simulink model "Boeing737Sample_updatedCopy"  (Simulink 8.2)
settings: Solver=ode45  StartTime=0.0  StopTime=100  RelTol=1e-3
InitFcn:
  | load('loss_coeff_mixing_junction.mat')
  | %load('defaultMSSN.mat')
  | load('SampleOutput.mat')
  | load('HydProp.mat')
  | load('HydraulicLoad.mat')
  | load('initavload.mat')
  | %load('mission_short.mat')
values from neighbouring files (symbols this model uses):
  avload =     [Benchmark_data1.mat]
  FuelBurn = [0 0 0 0 0 0 0 0 0 0 0 0 ... (18249 elements, 1x18249)]    [Benchmark_data1.mat]
undefined symbols (not defined in the file or in its folder): ailerons, B_737, elevator, F1, F2, HUGHES_TREITLER, landing_gear, PN_70147, rudder, thrust_rev
libraries: PowerFlowLib x91, simulink x19
(part 1 of 8)
settings Model: Creator=mwillms4  LastModifiedBy=srikanthan
settings DebuggingCC: FcnCallInpInsideContextMsg=EnableAllAsWarning  UnconnectedInputMsg=none  UnconnectedOutputMsg=none  UnconnectedLineMsg=none

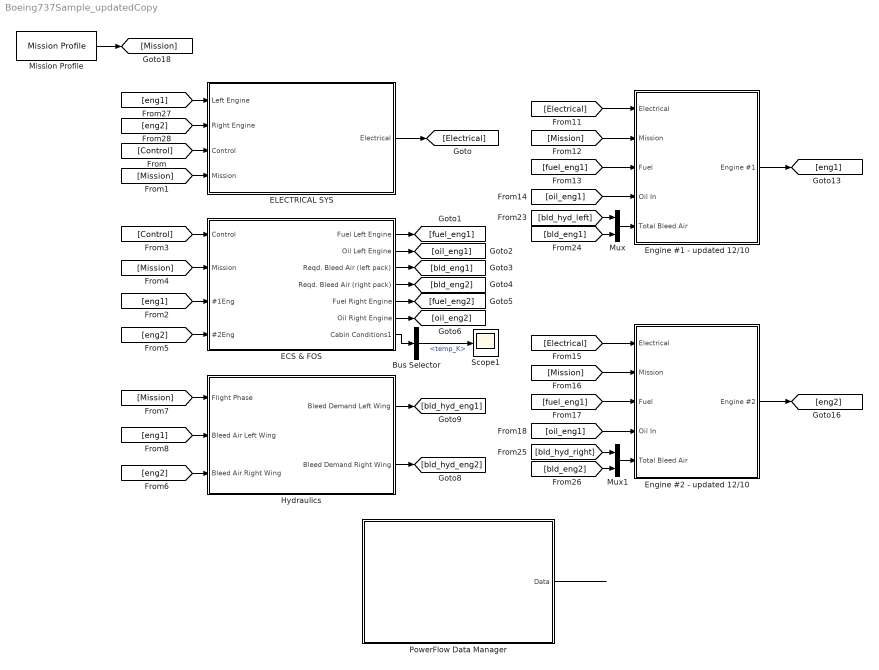
== system Boeing737Sample_updatedCopy ==
  Bus Selector : BusSelector  OutputSignals=temp_K
  "ECS & FOS " : Subsystem
  "ELECTRICAL SYS " : Subsystem
  Engine #1 - updated 12/10 : Subsystem
  Engine #2 - updated 12/10 : Subsystem
  "Hydraulics " : Subsystem
  Mission Profile : PowerFlowLib/Mission Profile/Mission Profile  mssn_check=off  mssn_prof=MSSN  del_P=0  del_T=0  del_rho=0  pres_msl=101.3  temp_msl=15  dens_msl=1.229
  Mux : Mux  Inputs=2
  Mux1 : Mux  Inputs=2
  PowerFlow Data Manager : Subsystem  AncestorBlock=PowerFlowLib/Support Functions//Tools/PowerFlow Data Manager
      mask init:
      | set_param(gcb, 'LinkStatus', 'inactive')    % disable the library link
      settings: OpenFcn=data_manager
      mask Display: str ='PowerFlow Data Manager\n(Double click to select variables for output)'; fprintf(str)
  Scope1 : Scope
      settings: YMin=295.065  YMax=295.075  SaveName=ScopeData36
  wires:
  Mission Profile/1 -> [Mission]
  "ELECTRICAL SYS "/1(Electrical) -> [Electrical]
  Engine #1 - updated 12/10/1(Engine #1) -> [eng1]
  Engine #2 - updated 12/10/1(Engine #2) -> [eng2]
  "Hydraulics "/2(Bleed Demand Right Wing) -> [bld_hyd_eng2]
  "Hydraulics "/1(Bleed Demand Left Wing) -> [bld_hyd_eng1]
  "ECS & FOS "/1("Fuel Left Engine ") -> [fuel_eng1]
  "ECS & FOS "/2(Oil Left Engine) -> [oil_eng1]
  "ECS & FOS "/3(Reqd. Bleed Air (left pack)) -> [bld_eng1]
  "ECS & FOS "/4(Reqd. Bleed Air (right pack)) -> [bld_eng2]
  "ECS & FOS "/5(Fuel Right Engine) -> [fuel_eng2]
  "ECS & FOS "/6(Oil Right Engine) -> [oil_eng2]
  [Mission] -> "Hydraulics "/1(Flight Phase)
  [eng2] -> "Hydraulics "/3(Bleed Air Right Wing)
  [eng1] -> "Hydraulics "/2(Bleed Air Left Wing)
  [Control] -> "ECS & FOS "/1(Control)
  [Mission] -> "ECS & FOS "/2(Mission)
  [Electrical] -> Engine #1 - updated 12/10/1(Electrical)
  [Mission] -> Engine #1 - updated 12/10/2(Mission)
  [fuel_eng1] -> Engine #1 - updated 12/10/3(Fuel)
  [oil_eng1] -> Engine #1 - updated 12/10/4(Oil In)
  [Electrical] -> Engine #2 - updated 12/10/1(Electrical)
  [Mission] -> Engine #2 - updated 12/10/2(Mission)
  [fuel_eng1] -> Engine #2 - updated 12/10/3(Fuel)
  [oil_eng1] -> Engine #2 - updated 12/10/4(Oil In)
  Mux/1 -> Engine #1 - updated 12/10/5(Total Bleed Air)
  [bld_eng1] -> Mux/2
  [bld_hyd_left] -> Mux/1
  Mux1/1 -> Engine #2 - updated 12/10/5(Total Bleed Air)
  [bld_eng2] -> Mux1/2
  [bld_hyd_right] -> Mux1/1
  Bus Selector/1 -> Scope1/1  "<temp_K>"
  [eng1] -> "ECS & FOS "/3(#1Eng)
  [eng2] -> "ECS & FOS "/4(#2Eng)
  PowerFlow Data Manager/1(Data) -> ?
  [Control] -> "ELECTRICAL SYS "/3(Control)
  [eng1] -> "ELECTRICAL SYS "/1(Left Engine)
  [eng2] -> "ELECTRICAL SYS "/2(Right Engine)
  [Mission] -> "ELECTRICAL SYS "/4(Mission)
  "ECS & FOS "/7(Cabin Conditions1) -> Bus Selector/1

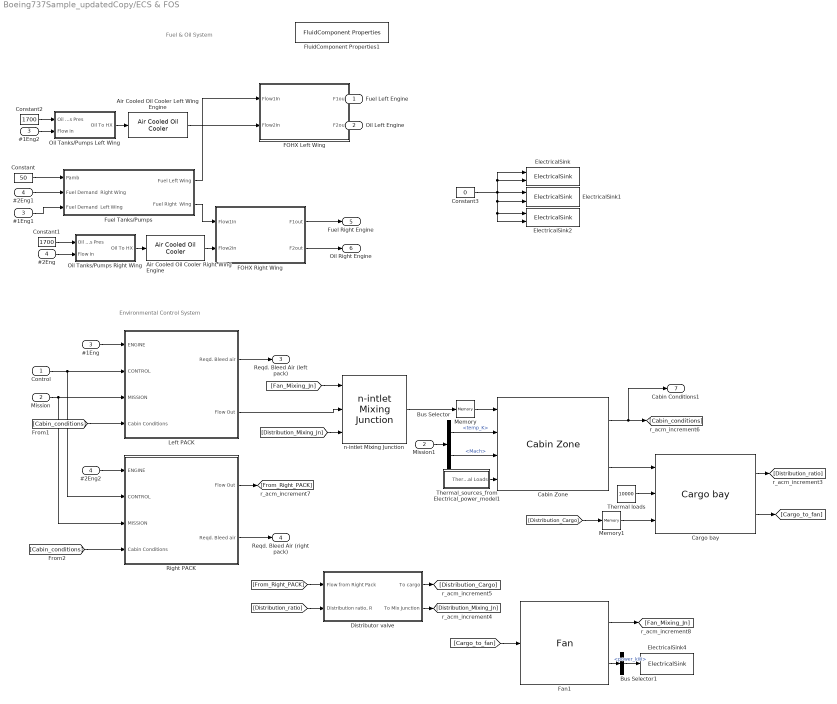
== system Boeing737Sample_updatedCopy/ECS & FOS  ==
  note: Environmental Control System
  note: Fuel & Oil System
  Control : Inport
  Mission : Inport  Port=2
  #1Eng : Inport  Port=3
  #2Eng : Inport  Port=4
  #1Eng1 : InportShadow  Port=3
  #1Eng2 : InportShadow  Port=3
  #2Eng1 : InportShadow  Port=4
  #2Eng2 : InportShadow  Port=4
  Air Cooled Oil Cooler Left Wing Engine : PowerFlowLib/Energy & Power Systems/Thermal/Oil/Air Cooled Oil Cooler  fileslct=off  filename=HeatExchangers.mat  filedir=C:\Users\mwillms4\Dropbox\School\Graduate\Research\PowerFlow Summer 2013\PropertyTables\HeatExchangers.mat  refresh=off  hx=HUGHES_TREITLER - PN_70147  bypass_full=1  bypass_none=100  hx_delP=82.74  hx_P=2068  hx_Qdot=24.27  hx_Vdot=0.000505  hx_mass=4.42
  Air Cooled Oil Cooler Right Wing Engine : PowerFlowLib/Energy & Power Systems/Thermal/Oil/Air Cooled Oil Cooler  fileslct=off  filename=HeatExchangers.mat  filedir=C:\Users\mwillms4\Dropbox\School\Graduate\Research\PowerFlow Summer 2013\PropertyTables\HeatExchangers.mat  refresh=off  hx=HUGHES_TREITLER - PN_70147  bypass_full=1  bypass_none=100  hx_delP=82.74  hx_P=2068  hx_Qdot=24.27  hx_Vdot=0.000505  hx_mass=4.42
  Bus Selector : BusSelector  OutputSignals=Flight parameters.temp_K,Flight parameters.Mach
  Bus Selector1 : BusSelector  OutputSignals=power_kW
  Cabin Zone : PowerFlowLib/Energy & Power Systems/Thermal/ECS/Cabin Zone  A_fuselage=320  V_cab=130.3  n_pass=176  L_shell=0.003  K_shell=1  L_insulation=0.02  K_insulation=1  L_coating=0.002  K_coating=1  Vdot_sa_pass=0.009438  q_pass=60  RAR=.25  h_outside=1  h_inside=1
  Cargo bay : PowerFlowLib/Energy & Power Systems/Thermal/ECS/Cargo bay  T_cargo_K=305
  Constant : Constant  Value=50
  Constant1 : Constant  Value=1700
  Constant2 : Constant  Value=1700
  Constant3 : Constant  Value=0
  Distributor valve : Subsystem
  ElectricalSink : PowerFlowLib/Support Functions//Tools/ElectricalSink  Tag=Flow  Description=TwoPhase  load_loc=Empennage  ACDC_load=AC  units=Kilowatts  unq_id=6691
  ElectricalSink1 : PowerFlowLib/Support Functions//Tools/ElectricalSink  Tag=Flow  Description=TwoPhase  load_loc=Cagobay  ACDC_load=AC  units=Kilowatts  unq_id=1878
  ElectricalSink2 : PowerFlowLib/Support Functions//Tools/ElectricalSink  Tag=Flow  Description=TwoPhase  load_loc=Cabin  ACDC_load=AC  units=Kilowatts  unq_id=3506
  ElectricalSink4 : PowerFlowLib/Support Functions//Tools/ElectricalSink  Tag=Flow  Description=TwoPhase  load_loc=Cabin  ACDC_load=DC  units=Kilowatts  unq_id=8332
  FOHX Left Wing : Subsystem  Description=TwoPhase  mask{fld1=JP8, fld2=LubeOil7808, alpha1=80, alpha2=80, N1=10, N2=10, A1_c=.1, A2_c=.1, A1_s=.25, A2_s=.25, P1init=620.5, P2init=620.5}
      mask prompts: fld1 "Fluid 1 Type"; fld2 "Fluid 2 Type"; alpha1 "Fluid 1 HTC [W/m² K]"; alpha2 "Fluid 2 HTC [W/m² K]"; N1 "Flow 1: Number of Channels"; N2 "Flow 2: Number of Channels"; A1_c "Flow 1: Cross-sectional area [m^2]"; A2_c "Flow 2: Cross-sectional area [m^2]"; A1_s "Flow 1: Total surface area [m^2]"; A2_s "Flow 2: Total surface area [m^2]"; P1init "Flow 1 Pressure [kPa]"; P2init "Flow 2 Pressure [kPa]"
      mask init:
      | %load TMSFluidProperties
      | %eval(['SF = FluidProp.SinglePhase.' get_param(gcb,'fld_type1') ';']);
      | %eval(['F = FluidProp.TwoPhase.' get_param(gcb,'fld_type2') ';']);
      | %FluidProp = FluidProp.TwoPhase.R134a; 
      | %{
      | if strcmp(get_param(bdroot,'SimulationStatus'),'initializing') ;
      |     load TwoPhaseProp_Evap
      |     TwoPhaseProp = TwoPhaseProp_Evap;
      |     Evaporator_Init_AFRL;
      | end
      | TMS_SetPhysSigs
      | if strcmp(get_param(gcb,'fld_type1'),'MoistAir')
      |     notair = 0 ; 
      | else
      |     notair = 1 ;
      | end
      | %}
      mask TypeOptions fld1: JP8
      mask TypeOptions fld2: LubeOil7808
      mask Display:
      | port_label('input',1,'Fuel In','TexMode','on') ;
      | port_label('input',2,'Oil In','TexMode','on') ;
      | port_label('output',1,'Fuel Out','TexMode','on') ;
      | port_label('output',2,'Oil Out','TexMode','on') ;
  FOHX Right Wing : Subsystem  Description=TwoPhase  mask{fld1=JP8, fld2=LubeOil7808, alpha1=80, alpha2=80, N1=10, N2=10, A1_c=.1, A2_c=.1, A1_s=.25, A2_s=.25, P1init=620.5, P2init=620.5}
      mask prompts: fld1 "Fluid 1 Type"; fld2 "Fluid 2 Type"; alpha1 "Fluid 1 HTC [W/m² K]"; alpha2 "Fluid 2 HTC [W/m² K]"; N1 "Flow 1: Number of Channels"; N2 "Flow 2: Number of Channels"; A1_c "Flow 1: Cross-sectional area [m^2]"; A2_c "Flow 2: Cross-sectional area [m^2]"; A1_s "Flow 1: Total surface area [m^2]"; A2_s "Flow 2: Total surface area [m^2]"; P1init "Flow 1 Pressure [kPa]"; P2init "Flow 2 Pressure [kPa]"
      mask init: same as Boeing737Sample_updatedCopy/ECS & FOS /FOHX Left Wing
      mask TypeOptions fld1: JP8
      mask TypeOptions fld2: LubeOil7808
      mask Display:
      | port_label('input',1,'Fuel In','TexMode','on') ;
      | port_label('input',2,'Oil In','TexMode','on') ;
      | port_label('output',1,'Fuel Out','TexMode','on') ;
      | port_label('output',2,'Oil Out','TexMode','on') ;
  Fan1 : PowerFlowLib/Energy & Power Systems/Thermal/ECS/Fan  N_fan=1725
  FluidComponent Properties1 : PowerFlowLib/Support Functions//Tools/FluidComponent Properties  fuelprop=FluidProp_JetA3638.mat  oilprop=OilProp.mat  airprop=AirProp.mat  pumpprop=PumpProp.mat  fanprop=Fanmap.mat  compprop=CompProp.mat  heatexprop=HeatExchangers.mat
  Fuel Tanks/Pumps : Subsystem
  Left PACK : Subsystem
  Memory : Memory
  Memory1 : Memory
  Mission1 : InportShadow  Port=2
  Oil Tanks/Pumps Left Wing : Subsystem
  Oil Tanks/Pumps Right Wing : Subsystem
  Right PACK : Subsystem
  Thermal loads : Constant  Value=10000
  Thermal_sources_from Electrical_power_model1 : Subsystem
  n-intlet Mixing Junction : PowerFlowLib/Energy & Power Systems/Thermal/ECS/n-intlet Mixing Junction  no_inlets=3  d_in_1=0.1  d_in_2=0.1  d_out=0.2
  "Fuel Left Engine " : Outport
  Oil Left Engine : Outport  Port=2
  Reqd. Bleed Air (left pack) : Outport  Port=3
  Reqd. Bleed Air (right pack) : Outport  Port=4
  Fuel Right Engine : Outport  Port=5
  Oil Right Engine : Outport  Port=6
  Cabin Conditions1 : Outport  Port=7
  wires:
  Left PACK/1(Reqd. Bleed air) -> Reqd. Bleed Air (left pack)/1
  Control/1 -> Left PACK/2(CONTROL), Right PACK/2(CONTROL)
  Mission/1 -> Left PACK/3(MISSION), Right PACK/3(MISSION)
  Right PACK/2(Reqd. Bleed air) -> Reqd. Bleed Air (right pack)/1
  Constant/1 -> Fuel Tanks/Pumps/1(Pamb)
  Air Cooled Oil Cooler Right Wing Engine/1 -> FOHX Right Wing/2(Flow2In)
  Fuel Tanks/Pumps/2(Fuel Right  Wing) -> FOHX Right Wing/1(Flow1In)
  Oil Tanks/Pumps Right Wing/1(Oil To HX) -> Air Cooled Oil Cooler Right Wing Engine/1
  Constant1/1 -> Oil Tanks/Pumps Right Wing/1(Oil Sys Pres)
  FOHX Right Wing/1(F1out) -> Fuel Right Engine/1
  Air Cooled Oil Cooler Left Wing Engine/1 -> FOHX Left Wing/2(Flow2In)
  Oil Tanks/Pumps Left Wing/1(Oil To HX) -> Air Cooled Oil Cooler Left Wing Engine/1
  Constant2/1 -> Oil Tanks/Pumps Left Wing/1(Oil Sys Pres)
  Fuel Tanks/Pumps/1(Fuel Left Wing) -> FOHX Left Wing/1(Flow1In)
  FOHX Left Wing/1(F1out) -> "Fuel Left Engine "/1
  FOHX Right Wing/2(F2out) -> Oil Right Engine/1
  FOHX Left Wing/2(F2out) -> Oil Left Engine/1
  Constant3/1 -> ElectricalSink1/1, ElectricalSink2/1, ElectricalSink2/2, ElectricalSink1/2, ElectricalSink/1, ElectricalSink/2
  n-intlet Mixing Junction/1 -> Memory/1
  Mission1/1 -> Bus Selector/1
  Bus Selector/1 -> Cabin Zone/2  "<temp_K>"
  Bus Selector/2 -> Cabin Zone/3  "<Mach>"
  Thermal_sources_from Electrical_power_model1/1(Thermal Loads) -> Cabin Zone/4
  Left PACK/2(Flow Out) -> n-intlet Mixing Junction/2
  Memory/1 -> Cabin Zone/1
  #1Eng2/1 -> Oil Tanks/Pumps Left Wing/2(Flow In)
  #2Eng1/1 -> Fuel Tanks/Pumps/2(Fuel Demand  Right Wing)
  #1Eng1/1 -> Fuel Tanks/Pumps/3(Fuel Demand  Left Wing)
  #2Eng/1 -> Oil Tanks/Pumps Right Wing/2(Flow In)
  #1Eng/1 -> Left PACK/1(ENGINE)
  #2Eng2/1 -> Right PACK/1(ENGINE)
  [Distribution_ratio] -> Distributor valve/2("Distribution ratio, R")
  [From_Right_PACK] -> Distributor valve/1(Flow from Right Pack)
  Distributor valve/2(To Mix Junction) -> [Distribution_Mixing_Jn]
  Distributor valve/1(To cargo) -> [Distribution_Cargo]
  Cabin Zone/1 -> Cabin Conditions1/1, [Cabin_conditions]
  [Fan_Mixing_Jn] -> n-intlet Mixing Junction/1
  [Cabin_conditions] -> Right PACK/4(Cabin Conditions)
  [Cabin_conditions] -> Left PACK/4(Cabin Conditions)
  Right PACK/1(Flow Out) -> [From_Right_PACK]
  [Distribution_Mixing_Jn] -> n-intlet Mixing Junction/3
  Bus Selector1/1 -> ElectricalSink4/1  "<power_kW>"
  [Cargo_to_fan] -> Fan1/1
  Fan1/1 -> [Fan_Mixing_Jn]
  Fan1/2 -> Bus Selector1/1
  [Distribution_Cargo] -> Memory1/1
  Cargo bay/1 -> [Distribution_ratio]
  Thermal loads/1 -> Cargo bay/2
  Memory1/1 -> Cargo bay/3
  Cabin Zone/2 -> Cargo bay/1
  Cargo bay/2 -> [Cargo_to_fan]

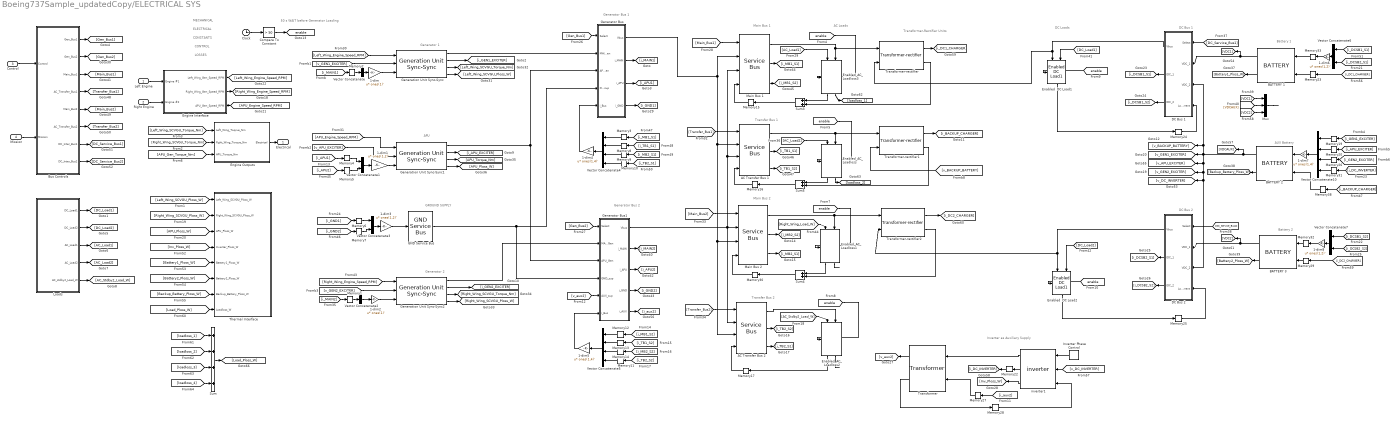
== system Boeing737Sample_updatedCopy/ELECTRICAL SYS  ==
  note: CONSTANTS
  note: CONTROL
  note: LOSSES
  note: MECHANICAL
  note: ELECTRICAL
  note: Generator Bus 1
  note: Generator 1
  note: APU
  note: GROUND SUPPLY
  note: Generator 2
  note: Main Bus 1
  note: Transfer Bus 1
  note: Main Bus 2
  note: Transfer Bus 2
  note: AC Loads
  note: Transformer-Rectifier Units
  note: DC Loads
  note: DC Bus 1
  note: DC Bus 2
  note: Battery 1
  note: AUX Battery
  note: Battery 2
  note: Inverter as Auxiliary Supply
  note: 50 s WAIT before Generator Loading
  note: Generator Bus 2
  Left Engine : Inport
  Right Engine : Inport  Port=2
  Control : Inport  Port=3
  Mission : Inport  Port=4
  " inverter1" : PowerFlowLib/Energy & Power Systems/Electrical/Inverters/ inverter  Trise=4e-6  Tfall=4e-6  fsw=2e3  Vcesat=1.2  Nofsw=6
  1-dim : Gain  Gain=ones(1)'  Multiplication=Matrix(u*K)
  1-dim{1,3,6,8} (4 alike) : Gain  Gain=ones(1,2)'  Multiplication=Matrix(u*K)
  1-dim2 : Gain  Gain=ones(1)'  Multiplication=Matrix(u*K)
  1-dim4 : Gain  Gain=ones(1,4)'  Multiplication=Matrix(u*K)
  1-dim5 : Gain  Gain=ones(1,4)'  Multiplication=Matrix(u*K)
  1-dim7 : Gain  Gain=ones(1,4)'  Multiplication=Matrix(u*K)
  AC Transfer Bus 1 : PowerFlowLib/Energy & Power Systems/Electrical/Systems/Service Bus
  AC Transfer Bus 2 : PowerFlowLib/Energy & Power Systems/Electrical/Systems/Service Bus
  BATTERY 1 : PowerFlowLib/Energy & Power Systems/Electrical/Battery/BATTERY  NO_CELLS=8  NO_MODULES=100  INITIAL_SOC=1
  BATTERY 2 : PowerFlowLib/Energy & Power Systems/Electrical/Battery/BATTERY  NO_CELLS=8  NO_MODULES=100  INITIAL_SOC=1
  BATTERY 3 : PowerFlowLib/Energy & Power Systems/Electrical/Battery/BATTERY  NO_CELLS=8  NO_MODULES=100  INITIAL_SOC=1
  Bus Controls : Subsystem  mask{BUS1=Generator 1, BUS2=Generator 2, MBUS1=Generator Bus 1, ACTBUS1=Generator Bus 1, MBUS2=Generator Bus 2, ACTBUS2=Generator Bus 2, IDCBUS1=Battery 1, IDCBUS2=Battery 2}
      mask prompts: BUS1 "Source for Bus 1"; BUS2 "Source for Bus 2"; MBUS1 "Load on Main Bus 1 drawn from"; ACTBUS1 "Load on AC Transfer Bus 1 drawn from"; MBUS2 "Load on Main Bus 2 drawn from"; ACTBUS2 "Load on AC Transfer Bus 2 drawn from"; IDCBUS1 "Source for DC Service Bus 1"; IDCBUS2 "Source for DC Service Bus 2"
      mask help:
      | Specify the source from which different buses receive power. There are
      | 1. Two Generator buses (Bus 1-2)
      | 2. Two AC Main buses (Main Bus 1-2))
      | 3. Two AC Transfer buses and (AC Transfer Bus 1-2)
      | 4. Two DC Intermediate buses (DC Intermediate Bus 1-2)
      mask init:
      | switch BUS1
      |     case 1
      |         BUS1CONTROL = 1;
      |     case 2
      |         BUS1CONTROL = 2;
      |     case 3
      |         BUS1CONTROL = 3;
      |     case 4
      |         BUS1CONTROL = 4;
      | end
      | 
      | switch BUS2
      |     case 1
      |         BUS2CONTROL = 1;
      |     case 2
      |         BUS2CONTROL = 2;
      |     case 3
      |         BUS2CONTROL = 3;
      |     case 4
      |         BUS2CONTROL = 4;
      | end
      | 
      | switch MBUS1
      |     case 1
      |         MBUS1CONTROL = 1;
      |     case 2
      |         MBUS1CONTROL = 2;
      | end
      | 
      | switch ACTBUS1
      |     case 1
      |         ACTBUS1CONTROL = 1;
      |     case 2
      |         ACTBUS1CONTROL = 2;
      | end
      | 
      | switch MBUS2
      |     case 1
      |         MBUS2CONTROL = 1;
      |     case 2
      |         MBUS2CONTROL = 2;
      | end
      | 
      | switch ACTBUS2
      |     case 1
      |         ACTBUS2CONTROL = 1;
      |     case 2
      |         ACTBUS2CONTROL = 2;
      | end
      | 
      | switch IDCBUS1
      |     case 1
      |         IDCBUS1CONTROL = 1;
      |     case 2
      |         IDCBUS1CONTROL = 2;
      | end
      | 
      | switch IDCBUS2
      |     case 1
      |         IDCBUS2CONTROL = 1;
      |     case 2
      |         IDCBUS2CONTROL = 2;
      | end
      mask TypeOptions BUS1: Generator 1  | APU  | GND | AUX SUPPLY
      mask TypeOptions BUS2: Generator 2  | APU  | GND | AUX SUPPLY
      mask TypeOptions MBUS1: Generator Bus 1 | Generator Bus 2
      mask TypeOptions ACTBUS1: Generator Bus 1 | Generator Bus 2
      mask TypeOptions MBUS2: Generator Bus 1 | Generator Bus 2
      mask TypeOptions ACTBUS2: Generator Bus 1 | Generator Bus 2
      mask TypeOptions IDCBUS1: Battery 1 | Battery 2
      mask TypeOptions IDCBUS2: Battery 1 | Battery 2
  Clock : Clock
  Compare To Constant : simulink/Logic and Bit Operations/Compare To Constant  relop=>  const=50  OutDataTypeStr=uint8
  DC Bus 1 : Subsystem  mask(DC Service Bus){}
      mask help: Service Bus
  DC Bus 2 : Subsystem  mask(DC Service Bus){}
      mask help: Service Bus
  Enabled  DC Load1 : PowerFlowLib/Energy & Power Systems/Electrical/Loads/Enabled  DC Load1
  Enabled  DC Load2 : PowerFlowLib/Energy & Power Systems/Electrical/Loads/Enabled  DC Load1
  Enabled_AC_Loadloss : PowerFlowLib/Energy & Power Systems/Electrical/Loads/Enabled_AC_Loadloss  P=0  Q=0  E=0.98  ILRMS=0  R=10000  X=10000
  Enabled_AC_Loadloss1 : PowerFlowLib/Energy & Power Systems/Electrical/Loads/Enabled_AC_Loadloss  P=0  Q=0  E=0.98  ILRMS=0  R=10000  X=10000
  Enabled_AC_Loadloss2 : PowerFlowLib/Energy & Power Systems/Electrical/Loads/Enabled_AC_Loadloss  P=0  Q=0  E=0.98  ILRMS=0  R=10000  X=10000
  Enabled_AC_Loadloss3 : PowerFlowLib/Energy & Power Systems/Electrical/Loads/Enabled_AC_Loadloss  P=500  Q=500  E=0.98  ILRMS=0  R=10000  X=10000
  Engine Interface : Subsystem
  Engine Outputs : Subsystem
  GND Service Bus : PowerFlowLib/Energy & Power Systems/Electrical/Systems/GND Service Bus
  Generation Unit Sync-Sync : PowerFlowLib/Energy & Power Systems/Electrical/Systems/Generation Unit Sync-Sync  machine_mode=300kVA_Gen  init_gear='init_gear_box.mat'  fan_load='init_fan_characteristics.mat'  exciter_param='exciter.mat'
  Generation Unit Sync-Sync1 : PowerFlowLib/Energy & Power Systems/Electrical/Systems/Generation Unit Sync-Sync  machine_mode=300kVA_Gen  init_gear='init_gear_box.mat'  fan_load='init_fan_characteristics.mat'  exciter_param='exciter.mat'
  Generation Unit Sync-Sync2 : PowerFlowLib/Energy & Power Systems/Electrical/Systems/Generation Unit Sync-Sync  machine_mode=300kVA_Gen  init_gear='init_gear_box.mat'  fan_load='init_fan_characteristics.mat'  exciter_param='exciter.mat'
  Generator Bus : Subsystem
      mask help: Generator Bus Structure.
  Generator Bus1 : Subsystem
      mask help: Generator Bus Structure.
  Inverter Phase Control : PowerFlowLib/Energy & Power Systems/Electrical/Systems/Inverter Phase Control
  Loads : Subsystem  mask(Avionics load configuration){avopt=Read from .mat file, mean=100, var=20, sampt=20, initavload='initavload.mat'}
      mask prompts: avopt "Enter Avionics load :"; mean "Mean load in W:"; var "Variance:"; sampt "Sample interval:"; initavload "Enter pathname of the mat file to load :"
      mask init:
      | blk = gcb;
      | value = get_param(blk,'avopt');
      | 
      | if strcmp(value,'As average with variation')
      |      STATS = 1;
      | else
      |      STATS = 2;
      |      load('initavload.mat');
      | end
      | 
      | clear blk value
      mask TypeOptions avopt: As average with variation | Read from .mat file
      mask Callback avopt:
      | blk = gcb;
      | value = get_param(blk,'avopt');
      | 
      | if strcmp(value,'As average with variation')
      |      STATS = 1;
      |      cellarr(1:4)={'on'};
      |      cellarr(5)={'off'};
      | else
      |      STATS = 2;
      |       cellarr(1)={'on'};
      |      cellarr(2:4)={'off'};
      |      cellarr(5)={'on'};
      |      load('initavload.mat');
      |  end
      |  set_param(blk,'MaskVisibilities',cellarr);
      |  clear blk STATS value cellarr
  Main Bus 1 : PowerFlowLib/Energy & Power Systems/Electrical/Systems/Service Bus
  Main Bus 2 : PowerFlowLib/Energy & Power Systems/Electrical/Systems/Service Bus
  Memory{1..17,19..20,22..33,38} (32 alike) : Memory
  Mux : Mux  Inputs=3
  Sum : Sum  Inputs=++++
  Sum3 : Sum
  Sum4 : Sum
  Sum5 : Sum
  Thermal Interface : Subsystem
  Transformer : PowerFlowLib/Energy & Power Systems/Electrical/Machines/Transformer  Rp=0.005  Rs=0.1  N1=32  N2=120
  Transformer-rectifier : PowerFlowLib/Energy & Power Systems/Electrical/Systems/Transformer-rectifier  pu=1
  Transformer-rectifier1 : PowerFlowLib/Energy & Power Systems/Electrical/Systems/Transformer-rectifier  pu=1
  Transformer-rectifier2 : PowerFlowLib/Energy & Power Systems/Electrical/Systems/Transformer-rectifier  pu=1
  Vector Concatenate : Concatenate  NumInputs=1  Mode=Multidimensional array  ConcatenateDimension=2
  Vector Concatenate{1,3,6..7} (4 alike) : Concatenate  Mode=Multidimensional array  ConcatenateDimension=2
  Vector Concatenate10 : Concatenate  NumInputs=4  Mode=Multidimensional array  ConcatenateDimension=2
  Vector Concatenate2 : Concatenate  NumInputs=1  Mode=Multidimensional array  ConcatenateDimension=2
  Vector Concatenate4 : Concatenate  NumInputs=4  Mode=Multidimensional array  ConcatenateDimension=2
  Vector Concatenate5 : Concatenate  NumInputs=4  Mode=Multidimensional array  ConcatenateDimension=2
  Electrical : Outport
  tag scope: enable=global
  wires:
  [AC_Stdby2_Load_W] -> Enabled_AC_Loadloss2/1
  AC Transfer Bus 2/1 -> Enabled_AC_Loadloss2/2
  Enabled_AC_Loadloss2/1 -> Memory17/1
  Memory17/1 -> AC Transfer Bus 2/4
  BATTERY 2/1 -> [v_GEN1_EXCITER], [v_APU_EXCITER], [v_GEN2_EXCITER], [v_DC_INVERTER], DC Bus 2/3(VDC_2), [v_BACKUP_BATTERY], DC Bus 1/3(VDC_2), [VDCAUX]
  BATTERY 3/1 -> DC Bus 2/2(VDC_1), [VDC2]
  BATTERY 1/1 -> DC Bus 1/2(VDC_1), [VDC1]
  Generation Unit Sync-Sync/1 -> Generator Bus/2(MAIN_Gen)
  GND Service Bus/1 -> Generator Bus/4(GND_sup), Generator Bus1/4(GND_sup)
  Generator Bus/3(i_APU) -> [i_APU1]
  Generator Bus/4(i_GND) -> [i_GND1]
  Vector Concatenate/1 -> 1-dim/1
  1-dim/1 -> Generation Unit Sync-Sync/3
  Vector Concatenate1/1 -> 1-dim1/1
  1-dim1/1 -> Generation Unit Sync-Sync1/3
  Vector Concatenate3/1 -> 1-dim3/1
  1-dim3/1 -> GND Service Bus/1
  [Left_Wing_Engine_Speed_RPM] -> Generation Unit Sync-Sync/1
  [APU_Engine_Speed_RPM] -> Generation Unit Sync-Sync1/1
  [Gen_Bus1] -> Generator Bus/1(Select)
  Generator Bus/1(Vbus) -> Main Bus 2/3, AC Transfer Bus 2/3, AC Transfer Bus 1/2, Main Bus 1/2
  [i_APU2] -> Memory5/1
  [i_GND2] -> Memory7/1
  Generation Unit Sync-Sync1/1 -> Generator Bus/3(APU_Gen), Generator Bus1/3(APU_Gen)
  [i_MAIN1] -> Memory2/1
  [i_APU1] -> Memory4/1
  [i_GND1] -> Memory6/1
  Memory2/1 -> Vector Concatenate/1
  Memory4/1 -> Vector Concatenate1/1
  Memory5/1 -> Vector Concatenate1/2
  Memory6/1 -> Vector Concatenate3/1
  Memory7/1 -> Vector Concatenate3/2
  Generator Bus/2(i_MAIN) -> [i_MAIN1]
  Generator Bus1/3(i_APU) -> [i_APU2]
  Generator Bus1/4(i_GND) -> [i_GND2]
  Generator Bus1/1(Vbus) -> Main Bus 1/3, AC Transfer Bus 1/3, Main Bus 2/2, AC Transfer Bus 2/2
  Generator Bus1/2(i_MAIN) -> [i_MAIN2]
  Vector Concatenate2/1 -> 1-dim2/1
  [i_MAIN2] -> Memory1/1
  Memory1/1 -> Vector Concatenate2/1
  Generation Unit Sync-Sync2/1 -> Generator Bus1/2(MAIN_Gen)
  [Gen_Bus2] -> Generator Bus1/1(Select)
  [Main_Bus1] -> Main Bus 1/1
  [Transfer_Bus1] -> AC Transfer Bus 1/1
  [Main_Bus2] -> Main Bus 2/1
  [Transfer_Bus2] -> AC Transfer Bus 2/1
  Main Bus 1/2 -> [i_MB1_S1]
  Main Bus 1/3 -> [i_MB1_S2]
  AC Transfer Bus 1/2 -> [i_TB1_S1]
  AC Transfer Bus 1/3 -> [i_TB1_S2]
  Main Bus 2/2 -> [i_MB2_S2]
  Main Bus 2/3 -> [i_MB2_S1]
  AC Transfer Bus 2/2 -> [i_TB2_S2]
  AC Transfer Bus 2/3 -> [i_TB2_S1]
  Main Bus 1/1 -> Transformer-rectifier/1, Enabled_AC_Loadloss3/2
  Memory15/1 -> Main Bus 1/4
  Memory16/1 -> AC Transfer Bus 1/4
  AC Transfer Bus 1/1 -> Transformer-rectifier1/1, Enabled_AC_Loadloss/2
  [AC_Load2] -> Enabled_AC_Loadloss/1
  Main Bus 2/1 -> Transformer-rectifier2/1, Enabled_AC_Loadloss1/2
  Memory30/1 -> Main Bus 2/4
  Generation Unit Sync-Sync/4 -> [Left_Wing_SCVGU_Ploss_W]
  Generation Unit Sync-Sync/3 -> [Left_Wing_SCVGU_Torque_Nm]
  Generation Unit Sync-Sync2/4 -> [Right_Wing_SCVGU_Ploss_W]
  Generation Unit Sync-Sync2/3 -> [Right_Wing_SCVGU_Torque_Nm]
  Generation Unit Sync-Sync1/3 -> [APU_Torque_Nm]
  Generation Unit Sync-Sync1/4 -> [APU_Ploss_W]
  [AC_Load1] -> Enabled_AC_Loadloss3/1
  [Right_Wing_Load_W] -> Enabled_AC_Loadloss1/1
  Engine Outputs/1(Electrical) -> Electrical/1
  [Left_Wing_SCVGU_Torque_Nm] -> Engine Outputs/1(Left_Wing_Toqrue_Nm)
  [Right_Wing_SCVGU_Torque_Nm] -> Engine Outputs/2(Rght_Wing_Torque_Nm)
  [APU_Gen_Torque_Nm] -> Engine Outputs/3(APU_Torque_Nm)
  Engine Interface/1(Left_Wing_Gen_Speed_RPM) -> [Left_Wing_Engine_Speed_RPM]
  Engine Interface/2(Right_Wing_Gen_Speed_RPM) -> [Right_Wing_Engine_Speed_RPM]
  Engine Interface/3(APU_Gen_Speed_RPM) -> [APU_Engine_Speed_RPM]
  DC Bus 1/1(Vbus) -> Transformer-rectifier/2, Enabled  DC Load1/1
  DC Bus 2/1(Vbus) -> Transformer-rectifier2/2, Enabled  DC Load2/1
  Memory24/1 -> DC Bus 1/4(Load current)
  Memory25/1 -> DC Bus 2/4(Load current)
  [DC_Service_Bus1] -> DC Bus 1/1(Select)
  [DC_Service_Bus2] -> DC Bus 2/1(Select)
  [DC_Load1] -> Enabled  DC Load1/2
  [DC_Load2] -> Enabled  DC Load2/2
  DC Bus 1/2(IDC_1) -> [i_DCSB1_S1]
  DC Bus 1/3(IDC_2) -> [i_DCSB1_S2]
  DC Bus 2/2(IDC_1) -> [i_DCSB2_S1]
  DC Bus 2/3(IDC_2) -> [i_DCSB2_S2]
  BATTERY 1/2 -> [Battery1_Ploss_W]
  BATTERY 2/2 -> [Backup_Battery_Ploss_W]
  BATTERY 3/2 -> [Battery2_Ploss_W]
  Left Engine/1 -> Engine Interface/1(Engine #1)
  Right Engine/1 -> Engine Interface/2(Engine #2)
  [v_GEN1_EXCITER] -> Generation Unit Sync-Sync/2
  Generation Unit Sync-Sync/2 -> [i_GEN1_EXCITER]
  [v_APU_EXCITER] -> Generation Unit Sync-Sync1/2
  Generation Unit Sync-Sync1/2 -> [i_APU_EXCITER]
  [Right_Wing_Engine_Speed_RPM] -> Generation Unit Sync-Sync2/1
  1-dim2/1 -> Generation Unit Sync-Sync2/3
  [v_GEN2_EXCITER] -> Generation Unit Sync-Sync2/2
  Generation Unit Sync-Sync2/2 -> [i_GEN2_EXCITER]
  Enabled  DC Load2/1 -> Memory25/1
  Memory27/1 -> Transformer/2
  Transformer-rectifier/2 -> Sum3/2
  Sum3/1 -> Memory15/1
  Enabled_AC_Loadloss3/1 -> Sum3/1
  Sum4/1 -> Memory30/1
  Enabled_AC_Loadloss1/1 -> Sum4/1
  Sum5/1 -> Memory16/1
  Enabled_AC_Loadloss/1 -> Sum5/1
  Transformer-rectifier1/1 -> [i_BACKUP_CHARGER]
  Clock/1 -> Compare To Constant/1
  Compare To Constant/1 -> [enable]
  [enable] -> Enabled_AC_Loadloss2/Enable
  [enable] -> Enabled  DC Load1/Enable
  [enable] -> Enabled  DC Load2/Enable
  Transformer/2 -> Memory28/1
  Transformer/1 -> [v_aux2]
  [v_aux2] -> Generator Bus1/5(AUX_sup)
  Generator Bus1/5(i_AUX) -> [i_aux2]
  " inverter1"/3 -> [Inv_Ploss_W]
  Memory28/1 -> " inverter1"/3
  " inverter1"/1 -> Transformer/1
  Inverter Phase Control/1 -> " inverter1"/1
  [v_DC_INVERTER] -> " inverter1"/2
  " inverter1"/2 -> Memory22/1
  Memory22/1 -> [i_DC_INVERTER]
  [i_aux2] -> Memory27/1
  [v_BACKUP_BATTERY] -> Transformer-rectifier1/2
  Transformer-rectifier1/2 -> Sum5/2
  Transformer-rectifier2/2 -> Sum4/2
  [enable] -> Enabled_AC_Loadloss/Enable
  [enable] -> Enabled_AC_Loadloss1/Enable
  [enable] -> Enabled_AC_Loadloss3/Enable
  Bus Controls/7(DC_Inter_Bus1) -> [DC_Service_Bus1]
  Bus Controls/8(DC_Inter_Bus2) -> [DC_Service_Bus2]
  Bus Controls/1(Gen_Bus1) -> [Gen_Bus1]
  Bus Controls/2(Gen_Bus2) -> [Gen_Bus2]
  Bus Controls/3(Main_Bus1) -> [Main_Bus1]
  Bus Controls/4(AC_Transfer_Bus1) -> [Transfer_Bus1]
  Bus Controls/5(Main_Bus2) -> [Main_Bus2]
  Bus Controls/6(AC_Transfer_Bus2) -> [Transfer_Bus2]
  Mission/1 -> Bus Controls/2(Mission)
  Control/1 -> Bus Controls/1(Control)
  Memory3/1 -> Vector Concatenate4/1
  Memory8/1 -> Vector Concatenate4/2
  Memory9/1 -> Vector Concatenate4/3
  Memory10/1 -> Vector Concatenate4/4
  [i_MB1_S1] -> Memory3/1
  [i_TB1_S1] -> Memory8/1
  [i_MB2_S1] -> Memory9/1
  [i_TB2_S1] -> Memory10/1
  Vector Concatenate4/1 -> 1-dim4/1
  1-dim4/1 -> Generator Bus/5(i_Bus)
  Memory12/1 -> Vector Concatenate5/1
  Memory13/1 -> Vector Concatenate5/2
  Memory14/1 -> Vector Concatenate5/3
  Memory11/1 -> Vector Concatenate5/4
  [i_MB1_S2] -> Memory12/1
  [i_TB1_S2] -> Memory13/1
  [i_MB2_S2] -> Memory14/1
  [i_TB2_S2] -> Memory11/1
  Vector Concatenate5/1 -> 1-dim5/1
  1-dim5/1 -> Generator Bus1/6(i_Bus)
  Loads/1(DC_Load1) -> [DC_Load1]
  Loads/2(DC_Load2) -> [DC_Load2]
  Loads/3(AC_Load1) -> [AC_Load1]
  Loads/4(AC_Load2) -> [AC_Load2]
  Loads/5(AC_stdby2_Load_W) -> [AC_Stdby2_Load_W]
  Memory33/1 -> BATTERY 1/1
  Memory23/1 -> BATTERY 1/2
  1-dim6/1 -> Memory33/1
  [i_DCSB1_S1] -> Vector Concatenate6/1
  [i_DCSB2_S1] -> Vector Concatenate6/2
  Vector Concatenate6/1 -> 1-dim6/1
  [i_DC1_CHARGER] -> Memory23/1
  Vector Concatenate10/1 -> 1-dim7/1
  1-dim7/1 -> BATTERY 2/1
  [i_GEN1_EXCITER] -> Memory19/1
  [i_APU_EXCITER] -> Memory20/1
  [i_GEN2_EXCITER] -> Memory26/1
  Memory38/1 -> BATTERY 2/2
  [i_BACKUP_CHARGER] -> Memory38/1
  Memory26/1 -> Vector Concatenate10/3
  Memory20/1 -> Vector Concatenate10/2
  Memory19/1 -> Vector Concatenate10/1
  Memory31/1 -> Vector Concatenate10/4
  [i_DC_INVERTER] -> Memory31/1
  Memory32/1 -> BATTERY 3/1
  1-dim8/1 -> Memory32/1
  [i_DCSB1_S2] -> Vector Concatenate7/1
  [i_DCSB2_S2] -> Vector Concatenate7/2
  Vector Concatenate7/1 -> 1-dim8/1
  Memory29/1 -> BATTERY 3/2
  [i_DC2_CHARGER] -> Memory29/1
  Transformer-rectifier/1 -> [i_DC1_CHARGER]
  Transformer-rectifier2/1 -> [i_DC2_CHARGER]
  Enabled  DC Load1/1 -> Memory24/1
  Mux/1 -> ?
  [VDC1] -> Mux/1
  [VDCAUX] -> Mux/2
  [VDC2] -> Mux/3
  [Left_Wing_SCVGU_Ploss_W] -> Thermal Interface/1(Left_Wing_SCVGU_Ploss_W)
  [Right_Wing_SCVGU_Ploss_W] -> Thermal Interface/2(Right_Wing_SCVGU_Ploss_W)
  [APU_Ploss_W] -> Thermal Interface/3(APU_Ploss_W)
  [Inv_Ploss_W] -> Thermal Interface/4(Inverter_Ploss_W)
  [Battery1_Ploss_W] -> Thermal Interface/5(Battery1_Ploss_W)
  [Battery2_Ploss_W] -> Thermal Interface/6(Battery2_Ploss_W)
  [Backup_Battery_Ploss_W] -> Thermal Interface/7(Backup_Battery_Ploss_W)
  [Load_Ploss_W] -> Thermal Interface/8(Loadloss_W)
  [loadloss_1] -> Sum/1
  [loadloss_2] -> Sum/2
  [loadloss_3] -> Sum/3
  [loadloss_4] -> Sum/4
  Sum/1 -> [Load_Ploss_W]
  Enabled_AC_Loadloss3/2 -> [loadloss_1]
  Enabled_AC_Loadloss/2 -> [loadloss_2]
  Enabled_AC_Loadloss1/2 -> ?
  Enabled_AC_Loadloss2/2 -> ?
